simulink model "test_memristor_zamarreno"  (R2018a)
settings: Solver=ode45  StartTime=0.0  StopTime=0.005  FixedStep=1e-4  MaxStep=1e-6  MinStep=1e-12  RelTol=1e-3  AbsTol=1e-6
libraries: fl_lib x5, nesl_utility x3, simulink x1
settings Model: Creator=bici  LastModifiedBy=bici
settings SolverCC: InitialStep=1e-10
settings DataIOCC: SaveState=on  InspectSignalLogs=on
settings SimscapeCC: SimscapeNormalizeSystem=off

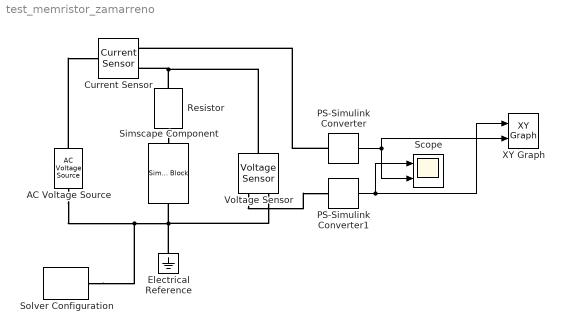
== system test_memristor_zamarreno ==
  AC Voltage Source : fl_lib/Electrical/Electrical Sources/AC Voltage Source  amp=2 V  shift=0 deg  frequency=1000 Hz  omega=0 rad/s
  Current Sensor : fl_lib/Electrical/Electrical Sensors/Current Sensor
      settings: LogSimulationData=on
  Electrical Reference : fl_lib/Electrical/Electrical Elements/Electrical Reference
  PS-Simulink Converter : nesl_utility/PS-Simulink Converter  PhysicalDomain=network_engine_domain  SubClassName=ps_output  LeftPortType=input  RightPortType=output  PseudoPeriodic=off  Frequencies=[]  Unit=1  AffineConversion=off
  PS-Simulink Converter1 : nesl_utility/PS-Simulink Converter  PhysicalDomain=network_engine_domain  SubClassName=ps_output  LeftPortType=input  RightPortType=output  PseudoPeriodic=off  Frequencies=[]  Unit=1  AffineConversion=off
  Resistor : fl_lib/Electrical/Electrical Elements/Resistor  R=5 MOhm  i_specify=off  i_priority=None  i=0 A  i_nominal_specify=off  i_nominal_unit=A  i_nominal_value=1  v_specify=off  v_priority=None  v=0 V  v_nominal_specify=off  v_nominal_unit=V  v_nominal_value=1
      settings: LogSimulationData=on
  Scope : Scope  NumInputPorts=2
  Simscape Component : SimscapeComponentBlock  SourceFile=memristor_zamarreno  ComponentPath=memristor_zamarreno  ComponentVariants=memristor_zamarreno  ComponentVariantNames=memristor_zamarreno  ClassName=memristor_zamarreno  SchemaVersion=1  Io=10 uA  Vo=0.1 V  Vth=1 V  x0=-9 V  Kr_inv=222 nA  w_max=10 V  w_min=-9 V  w_0=12.2 V  Cmr=10 mF  i_specify=off  i_priority=None  i=0 A  i_nominal_specify=off  i_nominal_unit=A  i_nominal_value=1  v_specify=off  v_priority=None  v=0 V  v_nominal_specify=off  v_nominal_unit=V  v_nominal_value=1
      settings: CopyFcn=simscape.engine.sli.internal.componentblockcallback(gcbh,'COPY')  PreCopyFcn=simscape.engine.sli.internal.componentblockcallback(gcbh,'PRECOPY')  PreDeleteFcn=simscape.engine.sli.internal.componentblockcallback(gcbh,'PREDELETE')  LogSimulationData=on
      mask Type: Zamarenov model memristora
  Solver Configuration : nesl_utility/Solver Configuration  PhysicalDomain=network_engine_domain  SubClassName=solver  LeftPortType=input  RightPortType=generic  Tones=[]  Harmonics=[]  SimulateNoise=off  Profile=off  UseLocalSampling=off  EnableSwitchedLinearOptims=on  FrequencyDomain=off  UseCCode=off  RelTol=0.001  AbsTol=1e-06  MinStep=1e-09  ToWorkspace=off  RevertToSquareIcSolve=off  NumHomotopyIterations=100  PhasorMode=off  PhasorModeNumHarmonics=1  DoDC=off  ResidualTolerance=1e-09  UseLocalSolver=off  LocalSolverChoice=NE_BACKWARD_EULER_ADVANCER  LocalSolverSampleTime=0.001  DoFixedCost=off  MaxNonlinIter=3  MaxModeIter=2  LinearAlgebra=Sparse  EquationFormulation=NE_TIME_EF  DelaysMemoryBudget=1024  AutomaticFiltering=on  FilteringTimeConstant=0.001
  Voltage Sensor : fl_lib/Electrical/Electrical Sensors/Voltage Sensor
  XY Graph : simulink/Sinks/XY Graph  xmin=-2.1  xmax=2.1  ymin=-150e-9  ymax=150e-9  st=-1
  wires:
  PS-Simulink Converter/1 -> Scope/2, XY Graph/2
  PS-Simulink Converter1/1 -> Scope/1, XY Graph/1
  connections:
  Solver Configuration/RConn1 -- AC Voltage Source/RConn1 -- Voltage Sensor/RConn2 -- Simscape Component/RConn1 -- Electrical Reference/LConn1
  Resistor/LConn1 -- Voltage Sensor/LConn1 -- Current Sensor/RConn2
  PS-Simulink Converter/LConn1 -- Current Sensor/RConn1
  Voltage Sensor/RConn1 -- PS-Simulink Converter1/LConn1
  AC Voltage Source/LConn1 -- Current Sensor/LConn1
  Resistor/RConn1 -- Simscape Component/LConn1
